simulink model "Sterowanie_StatkiemDEDI_2015"  (R2015b)
settings: Solver=FixedStepAuto  SolverMode=SingleTasking  StartTime=0.0  StopTime=10  FixedStep=0.001  MaxStep=0.01  MinStep=.009  RelTol=1e-2
settings Model: Creator=szymo  LastModifiedBy=szymo
settings SolverCC: AlgebraicLoopSolver=LineSearch
settings DataIOCC: LimitDataPoints=off  ReturnWorkspaceOutputs=on
settings DebuggingCC: AllowSymbolicDim=on  SFUnexpectedBacktrackingDiag=error  SFNoUnconditionalDefaultTransitionDiag=error
settings ModelReferenceCC: PropagateSignalLabelsOutOfModel=on
settings SFSimCC: SimUseLocalCustomCode=on
settings RTWCC: RTWUseLocalCustomCode=on
settings GRTTargetCC: TargetLangStandard=C99 (ISO)
settings ConfigComp: CovMetricSettings=dwe  CovHtmlReporting=off  CovSaveCumulativeToWorkspaceVar=off  CovSaveSingleToWorkspaceVar=off  CovModelRefEnable=Off  CovExternalEMLEnable=on

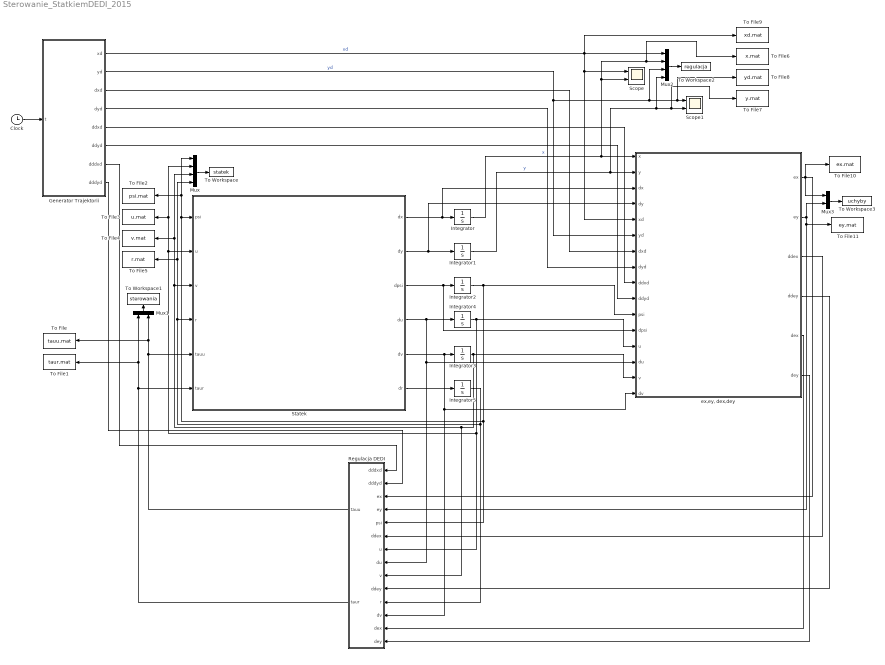
== system Sterowanie_StatkiemDEDI_2015 ==
  Clock : Clock
  Generator Trajektorii : MATLAB Function  TreatAsAtomicUnit=on
  Integrator : Integrator  InitialCondition=-0.01
  Integrator1 : Integrator  InitialCondition=1.01
  Integrator2 : Integrator  InitialCondition=0.01
  Integrator3 : Integrator  InitialCondition=0.1
  Integrator4 : Integrator  InitialCondition=0.1
  Integrator5 : Integrator  InitialCondition=0.1
  Mux : Mux
  Mux1 : Mux  Inputs=2
  Mux2 : Mux
  Mux3 : Mux  Inputs=2
  Regulacja DEDI : Subsystem
  Scope : Scope  NumInputPorts=2
  Scope1 : Scope  NumInputPorts=2
  Statek : MATLAB Function  TreatAsAtomicUnit=on
  To File : ToFile  Filename=tauu.mat  SaveFormat=Timeseries
  To File1 : ToFile  Filename=taur.mat  SaveFormat=Timeseries
  To File10 : ToFile  Filename=ex.mat  SaveFormat=Timeseries
  To File11 : ToFile  Filename=ey.mat  SaveFormat=Timeseries
  To File2 : ToFile  Filename=psi.mat  SaveFormat=Timeseries
  To File3 : ToFile  Filename=u.mat  SaveFormat=Timeseries
  To File4 : ToFile  Filename=v.mat  SaveFormat=Timeseries
  To File5 : ToFile  Filename=r.mat  SaveFormat=Timeseries
  To File6 : ToFile  Filename=x.mat  SaveFormat=Timeseries
  To File7 : ToFile  Filename=y.mat  SaveFormat=Timeseries
  To File8 : ToFile  Filename=yd.mat  SaveFormat=Timeseries
  To File9 : ToFile  Filename=xd.mat  SaveFormat=Timeseries
  To Workspace : ToWorkspace  VariableName=statek  SaveFormat=Timeseries  SampleTime=-1
  To Workspace1 : ToWorkspace  VariableName=sterowania  SaveFormat=Timeseries  SampleTime=-1
  To Workspace2 : ToWorkspace  VariableName=regulacja  SaveFormat=Timeseries  SampleTime=-1
  To Workspace3 : ToWorkspace  VariableName=uchyby  SaveFormat=Timeseries  SampleTime=-1
  "ex,ey, dex,dey" : MATLAB Function  TreatAsAtomicUnit=on
  wires:
  Clock/1 -> Generator Trajektorii/1(t)
  Statek/1(dx) -> "ex,ey, dex,dey"/3(dx), Integrator/1
  Statek/2(dy) -> Integrator1/1, "ex,ey, dex,dey"/4(dy)
  Statek/3(dpsi) -> "ex,ey, dex,dey"/12(dpsi), Integrator2/1
  Statek/4(du) -> Regulacja DEDI/8(du), "ex,ey, dex,dey"/14(du), Integrator4/1
  Statek/5(dv) -> Regulacja DEDI/12(dv), "ex,ey, dex,dey"/16(dv), Integrator3/1
  Statek/6(dr) -> Integrator5/1
  Integrator2/1 -> "ex,ey, dex,dey"/11(psi), Regulacja DEDI/5(psi), To File2/1, Mux/1, Statek/1(psi)
  Integrator4/1 -> "ex,ey, dex,dey"/13(u), Regulacja DEDI/7(u), To File3/1, Mux/2, Statek/2(u)
  Integrator5/1 -> Regulacja DEDI/11(r), To File5/1, Mux/4, Statek/4(r)
  Integrator/1 -> "ex,ey, dex,dey"/1(x), To File6/1, Mux2/2, Scope/2  "x"
  Integrator1/1 -> Mux2/4, To File7/1, Scope1/2, "ex,ey, dex,dey"/2(y)  "y"
  Generator Trajektorii/1(xd) -> Scope/1, "ex,ey, dex,dey"/5(xd), Mux2/1, To File9/1  "xd"
  Generator Trajektorii/2(yd) -> Mux2/3, To File8/1, Scope1/1, "ex,ey, dex,dey"/6(yd)  "yd"
  Generator Trajektorii/5(ddxd) -> "ex,ey, dex,dey"/9(ddxd)
  Generator Trajektorii/6(ddyd) -> "ex,ey, dex,dey"/10(ddyd)
  Generator Trajektorii/3(dxd) -> "ex,ey, dex,dey"/7(dxd)
  Generator Trajektorii/4(dyd) -> "ex,ey, dex,dey"/8(dyd)
  Regulacja DEDI/2(taur) -> To File1/1, Mux1/1, Statek/6(taur)
  Generator Trajektorii/7(dddxd) -> Regulacja DEDI/1(dddxd)
  Generator Trajektorii/8(dddyd) -> Regulacja DEDI/2(dddyd)
  "ex,ey, dex,dey"/1(ex) -> To File10/1, Mux3/1, Regulacja DEDI/3(ex)
  "ex,ey, dex,dey"/2(ey) -> Mux3/2, To File11/1, Regulacja DEDI/4(ey)
  "ex,ey, dex,dey"/3(ddex) -> Regulacja DEDI/6(ddex)
  Integrator3/1 -> Regulacja DEDI/9(v), To File4/1, Mux/3, Statek/3(v), "ex,ey, dex,dey"/15(v)
  "ex,ey, dex,dey"/4(ddey) -> Regulacja DEDI/10(ddey)
  "ex,ey, dex,dey"/5(dex) -> Regulacja DEDI/13(dex)
  "ex,ey, dex,dey"/6(dey) -> Regulacja DEDI/14(dey)
  Mux/1 -> To Workspace/1
  Mux1/1 -> To Workspace1/1
  Mux2/1 -> To Workspace2/1
  Mux3/1 -> To Workspace3/1
  Regulacja DEDI/1(tauu) -> Statek/5(tauu), To File/1, Mux1/2

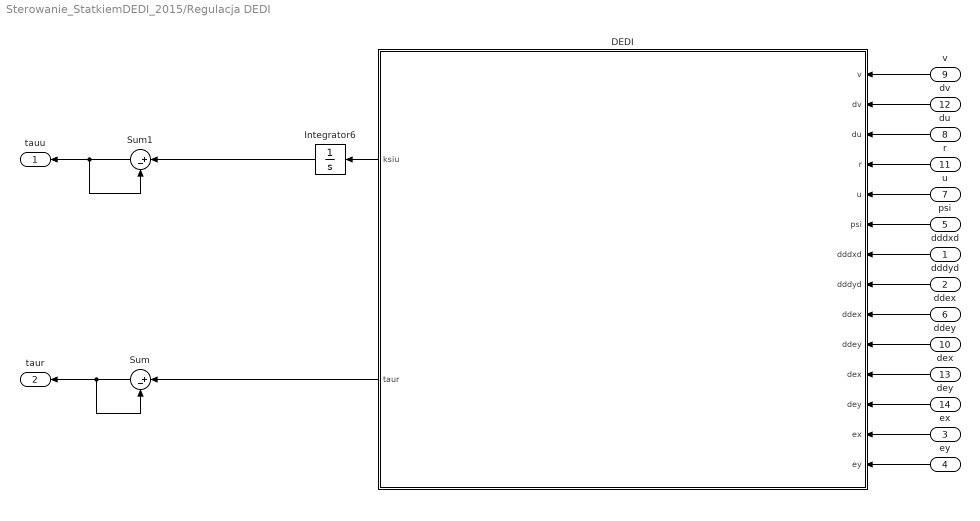
== system Sterowanie_StatkiemDEDI_2015/Regulacja DEDI ==
  dddxd : Inport
  dddyd : Inport  Port=2
  ex : Inport  Port=3
  ey : Inport  Port=4
  psi : Inport  Port=5
  ddex : Inport  Port=6
  u : Inport  Port=7
  du : Inport  Port=8
  v : Inport  Port=9
  ddey : Inport  Port=10
  r : Inport  Port=11
  dv : Inport  Port=12
  dex : Inport  Port=13
  dey : Inport  Port=14
  DEDI : MATLAB Function  TreatAsAtomicUnit=on
  Integrator6 : Integrator
  Sum : Sum  Inputs=|+-
  Sum1 : Sum  Inputs=|+-
  tauu : Outport
  taur : Outport  Port=2
  wires:
  DEDI/1(ksiu) -> Integrator6/1
  Sum/1 -> Sum/2, taur/1
  ex/1 -> DEDI/13(ex)
  ddex/1 -> DEDI/9(ddex)
  ddey/1 -> DEDI/10(ddey)
  du/1 -> DEDI/3(du)
  dv/1 -> DEDI/2(dv)
  ey/1 -> DEDI/14(ey)
  u/1 -> DEDI/5(u)
  psi/1 -> DEDI/6(psi)
  Sum1/1 -> Sum1/2, tauu/1
  r/1 -> DEDI/4(r)
  dddxd/1 -> DEDI/7(dddxd)
  dddyd/1 -> DEDI/8(dddyd)
  v/1 -> DEDI/1(v)
  dex/1 -> DEDI/11(dex)
  dey/1 -> DEDI/12(dey)
  Integrator6/1 -> Sum1/1
  DEDI/2(taur) -> Sum/1

== matlab function Sterowanie_StatkiemDEDI_2015/Generator Trajektorii ==
  data: t input; xd output; yd output; dxd output; dyd output; ddxd output; ddyd output; dddxd output; dddyd output
function [xd,yd,dxd,dyd,ddxd,ddyd,dddxd,dddyd] = fcn(t)

xd = sin(t);
yd = cos(t);
dxd=cos(t);
dyd=-sin(t);
ddxd = -sin(t);
ddyd = -cos(t);
dddxd = -cos(t);
dddyd = sin(t);

== matlab function Sterowanie_StatkiemDEDI_2015/Statek ==
  data: psi input size=1; u input size=1; v input size=1; dx output size=1; r input size=1; dy output size=1; dpsi output size=1; du output size=1; dv output size=1; dr output size=1; tauu input size=1; taur input size=1
function [dx,dy,dpsi,du,dv,dr] = fcn(psi,u,v,r,tauu,taur)
m11=1.956;
m22=2.405;
m33=0.043;
d11=2.436;
d22=12.992;
d33=0.0564;
dx = u*cos(psi)-v*sin(psi);
dy = u*sin(psi)+v*cos(psi);
dpsi = r;
du = (m22*v*r-d11*u+tauu)/m11;
dv = (-m11*u*r-d22*v)/m22;
dr = ((m11-m22)*u*v-d33*r+taur)/m33;

== matlab function Sterowanie_StatkiemDEDI_2015/ex,ey, dex,dey ==
  data: x input; y input; dx input; dy input; xd input; yd input; dxd input; dyd input; ddxd input; ddyd input; psi input; dpsi input; u input; du input; v input; dv input; ex output; ey output; ddex output; ddey output; dex output; dey output
function [ex,ey,ddex,ddey,dex,dey] = fcn(x,y,dx,dy,xd,yd,dxd,dyd,ddxd,ddyd,psi,dpsi,u,du,v,dv)

ex = x-xd;
ey = y-yd;
m11=1.956;
dex=dx-dxd;
dey=dy-dyd;
ddex = du*cos(psi)-u*dpsi*sin(psi)-dv*sin(psi)-v*dpsi*cos(psi)-ddxd;
ddey = du*sin(psi)+u*dpsi*cos(psi)+dv*cos(psi)-v*dpsi*sin(psi)-ddyd;

== matlab function Sterowanie_StatkiemDEDI_2015/Regulacja DEDI/DEDI ==
  data: v input; dv input; du input; r input; u input; ksiu output; psi input; dddxd input; dddyd input; ddex input; ddey input; dex input; dey input; ex input; ey input; taur output
function [ksiu,taur] = fcn(v,dv,du,r,u,psi,dddxd,dddyd,ddex,ddey,dex,dey,ex,ey)

m11=1.956;
m22=2.405;
m33=0.043;
d11=2.436;
d22=12.992;
d33=0.0564;

k11=6;
k12=12;
k13=8;
k14=6;
k15=12;
k16=8;

%fu = (m22*v*r-d11*u)/m11;
fr = ((m11-m22)*u*v-d33*r)/m33;
%gu = 1/m11;
%gr = 1/m33;

au = (m22*dv*r+m22*v*fr-d11*du)/m11;
av = (-m11*du*r-m11*u*fr-d22*dv)/m22;
%bu = m22*v/(m11*m33);
%bv = -m11*u/(m22*m33);

F1 = [(au-2*dv*r-v*fr-u*r^2)*cos(psi)-(av+2*du*r+u*fr-v*r^2)*sin(psi)-dddxd; (au-2*dv*r-v*fr-u*r^2)*sin(psi)+(av+2*du*r+u*fr-v*r^2)*cos(psi)-dddyd];
G1 = [cos(psi)/m11, ((m22/m11-1)*v*cos(psi)+(m11/m22-1)*u*sin(psi))/m33; sin(psi)/m11, ((m22/m11-1)*v*sin(psi)+(1-m11/m22)*u*cos(psi))/m33];


wek = G1^(-1)*(-1*F1+[-k11*ddex-k12*dex-k13*ex;-k14*ddey-k15*dey-k16*ey]);
ksiu = wek(1);
taur = wek(2);
